simulink model "simulation_basic"  (R2022b)
settings: Solver=ode4  StartTime=0.0  StopTime=10  FixedStep=5e-7  MaxStep=1e-6  RelTol=1e-3
undefined symbols (not defined in the file or in its folder): current, Down, inverter, motor, speed, Up
libraries: simulink x11, eeGeneralControl x7, mcbcontrolslib x5, slpidlib x3, SignalEditorBlockLib x2, spsTriangleGeneratorLib x2, spsSampleandHoldLib x1
(part 1 of 2)
settings Model: Creator=Rizwan Sadik  LastModifiedBy=Rizwan Sadik
settings DataIOCC: SaveOutput=off  SaveTime=off

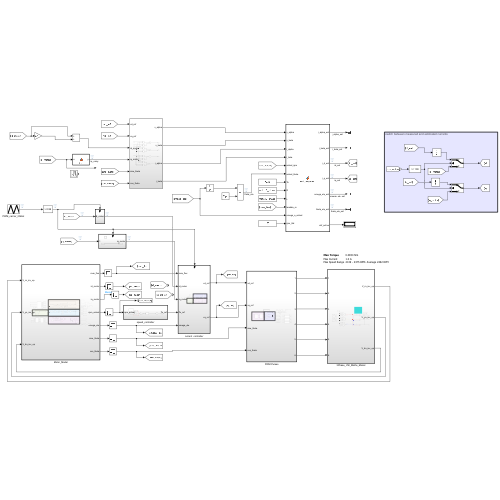
[thumbnail: Simulink's stored preview of the top-level diagram]
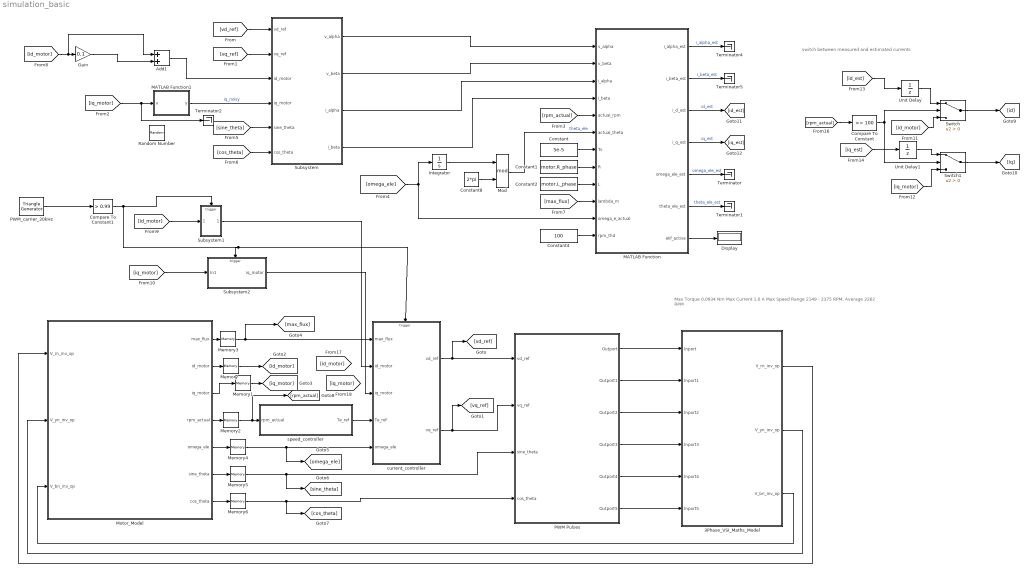
== system simulation_basic ==
  note: switch between measured and estimated currents
  note: Max Torque
      | 0.0934 Nm
      |
      | Max Current
      | 1.0 A
      |
      | Max Speed Range
      | 2149 - 2375 RPM. Average 2262 RPM
  3Phase_VSI_Maths_Model : Subsystem  Description=|  TreatAsAtomicUnit=on
      | Input DC Voltage = Vdc
      | Ouput Phase Voltages = Vrn, Vyn, Vbn
      | 
      | Pole Voltage = Vdc/2
      | Pole Voltages - instantaneous values:
      | Vro = +- Vdc/2
      | Vyo = +- Vdc/2
      | Vbo = +- Vdc/2
      | 
      | Leg 1 o/p is Vr. Switches 1 & 4
      | sw 1 ON (sw 4 OFF) -> Vro = +Vdc/2
      | sw 4 ON (sw 1 OFF) -> Vro = -Vdc/2
      | 
      | Leg 2 o/p is Vy. Switches 3 & 6
      | sw 3 ON (sw 6 OFF) -> Vyo = +Vdc/2
      | sw 6 ON (sw 3 OFF) -> Vyo = -Vdc/2
      | 
      | Leg 3 o/p is Vb. Switches 5 & 2
      | sw 5 ON (sw 2 OFF) -> Vbo = +Vdc/2
      | sw 2 ON (sw 5 OFF) -> Vbo = -Vdc/2
      | 
      | Vrn = (2Vro-Vyo-Vbo)/3
      | Vyn = (2Vyo-Vro-Vbo)/3
      | Vbn =(2Vbo-Vyo-Vro)/3
  Add1 : Sum
  Compare To Constant : simulink/Logic and Bit Operations/Compare To Constant  relop=>=  const=100  OutDataTypeStr=boolean
  Compare To Constant1 : simulink/Logic and Bit Operations/Compare To Constant  relop=>  const=0.99  OutDataTypeStr=boolean
  Constant : Constant  Value=5e-5
  Constant1 : Constant  Value=motor.R_phase
  Constant2 : Constant  Value=motor.L_phase
  Constant4 : Constant  Value=100
  Constant8 : Constant  Value=2*pi
  Display : Display
  Gain : Gain  Gain=0.1
  Integrator : Integrator  WrappedStateUpperValue=2*pi  WrappedStateLowerValue=0
  MATLAB Function : MATLAB Function  TreatAsAtomicUnit=on
  MATLAB Function1 : MATLAB Function  TreatAsAtomicUnit=on
  Memory{,1..6} (7 alike) : Memory
  Mod : Math  Operator=mod
  Motor_Model : Subsystem  TreatAsAtomicUnit=on
  PWM Pulses : Subsystem  TreatAsAtomicUnit=on
  PWM_carrier_20kHz : spsTriangleGeneratorLib/Triangle Generator  Freq=20000  Phase=0  Ts=0
  Random Number : RandomNumber  SampleTime=0.1
  Subsystem : Subsystem
  Subsystem1 : Subsystem
  Subsystem2 : Subsystem
  Switch : Switch  Criteria=u2 > Threshold  SaturateOnIntegerOverflow=off  InputSameDT=off
  Switch1 : Switch  Criteria=u2 > Threshold  SaturateOnIntegerOverflow=off  InputSameDT=off
  Terminator{,1..2,4..5} (5 alike) : Terminator
  Unit Delay : UnitDelay  SampleTime=-1  HasFrameUpgradeWarning=on
  Unit Delay1 : UnitDelay  SampleTime=-1  HasFrameUpgradeWarning=on
  current_controller : Subsystem  TreatAsAtomicUnit=on
  speed_controller : Subsystem  TreatAsAtomicUnit=on
  wires:
  speed_controller/1(Te_ref) -> current_controller/4(Te_ref)
  PWM Pulses/1(Outport) -> 3Phase_VSI_Maths_Model/1(Inport)
  Motor_Model/1(max_flux) -> Memory3/1
  PWM Pulses/4(Outport3) -> 3Phase_VSI_Maths_Model/4(Inport3)
  PWM Pulses/5(Outport4) -> 3Phase_VSI_Maths_Model/5(Inport4)
  Motor_Model/6(sine_theta) -> Memory5/1
  PWM Pulses/3(Outport2) -> 3Phase_VSI_Maths_Model/3(Inport2)
  Motor_Model/3(iq_motor) -> Memory1/1
  PWM Pulses/2(Outport1) -> 3Phase_VSI_Maths_Model/2(Inport1)
  PWM Pulses/6(Outport5) -> 3Phase_VSI_Maths_Model/6(Inport5)
  Motor_Model/2(id_motor) -> Memory/1
  Motor_Model/7(cos_theta) -> Memory6/1
  current_controller/2(vq_ref) -> [vq_ref], PWM Pulses/2(vq_ref)
  current_controller/1(vd_ref) -> [vd_ref], PWM Pulses/1(vd_ref)
  3Phase_VSI_Maths_Model/3(V_bn_inv_op) -> Motor_Model/3(V_bn_inv_op)
  3Phase_VSI_Maths_Model/2(V_yn_inv_op) -> Motor_Model/2(V_yn_inv_op)
  3Phase_VSI_Maths_Model/1(V_rn_inv_op) -> Motor_Model/1(V_rn_inv_op)
  Motor_Model/4(rpm_actual) -> Memory2/1
  Subsystem/3(i_alpha) -> MATLAB Function/3(i_alpha)
  Subsystem/4(i_beta) -> MATLAB Function/4(i_beta)
  Constant/1 -> MATLAB Function/7(Ts)
  Constant1/1 -> MATLAB Function/8(R)
  Constant2/1 -> MATLAB Function/9(L)
  MATLAB Function/5(omega_ele_est) -> Terminator/1  "omega_ele_est"
  MATLAB Function/6(theta_ele_est) -> Terminator1/1  "theta_ele_est"
  Motor_Model/5(omega_ele) -> Memory4/1
  Constant4/1 -> MATLAB Function/12(rpm_thd)
  MATLAB Function/7(ekf_active) -> Display/1
  Mod/1 -> MATLAB Function/6(actual_theta)  "theta_ele"
  Constant8/1 -> Mod/2
  Integrator/1 -> Mod/1
  Subsystem/1(v_alpha) -> MATLAB Function/1(v_alpha)
  Subsystem/2(v_beta) -> MATLAB Function/2(v_beta)
  [omega_ele] -> MATLAB Function/11(omega_e_actual), Integrator/1
  MATLAB Function/3(i_d_est) -> [id_est]  "id_est"
  MATLAB Function/4(i_q_est) -> [iq_est]  "iq_est"
  [vd_ref] -> Subsystem/1(vd_ref)
  [vq_ref] -> Subsystem/2(vq_ref)
  [id_motor] -> Add1/1, Gain/1
  [iq_motor] -> Terminator2/1, MATLAB Function1/1(u)
  [sine_theta] -> Subsystem/5(sine_theta)
  [cos_theta] -> Subsystem/6(cos_theta)
  [max_flux] -> MATLAB Function/10(lambda_m)
  [rpm_actual] -> MATLAB Function/5(actual_rpm)
  MATLAB Function/2(i_beta_est) -> Terminator5/1  "i_beta_est"
  MATLAB Function/1(i_alpha_est) -> Terminator4/1  "i_alpha_est"
  Subsystem1/1(id_motor) -> current_controller/2(id_motor)
  Subsystem2/1(iq_motor) -> current_controller/3(iq_motor)
  Switch/1 -> [id]
  Switch1/1 -> [iq]
  [id_motor] -> Switch/3
  [iq_motor] -> Switch1/3
  [id_est] -> Unit Delay/1
  [iq_est] -> Unit Delay1/1
  [rpm_actual] -> Compare To Constant/1
  Compare To Constant/1 -> Switch1/2, Switch/2
  Unit Delay/1 -> Switch/1
  Unit Delay1/1 -> Switch1/1
  Memory/1 -> [id_motor]
  Memory1/1 -> [iq_motor]
  Memory2/1 -> [rpm_actual], speed_controller/1(rpm_actual)
  Memory3/1 -> [max_flux], current_controller/1(max_flux)
  Memory4/1 -> [omega_ele], current_controller/5(omega_ele)
  Memory5/1 -> [sine_theta], PWM Pulses/3(sine_theta)
  Memory6/1 -> [cos_theta], PWM Pulses/4(cos_theta)
  Gain/1 -> Add1/2
  Add1/1 -> Subsystem/3(id_motor)
  MATLAB Function1/1(y) -> Subsystem/4(iq_motor)  "iq_noisy"
  PWM_carrier_20kHz/1 -> Compare To Constant1/1
  Compare To Constant1/1 -> current_controller/Trigger, Subsystem2/Trigger, Subsystem1/Trigger
  [id_motor] -> Subsystem1/1(In1)
  [iq_motor] -> Subsystem2/1(In1)

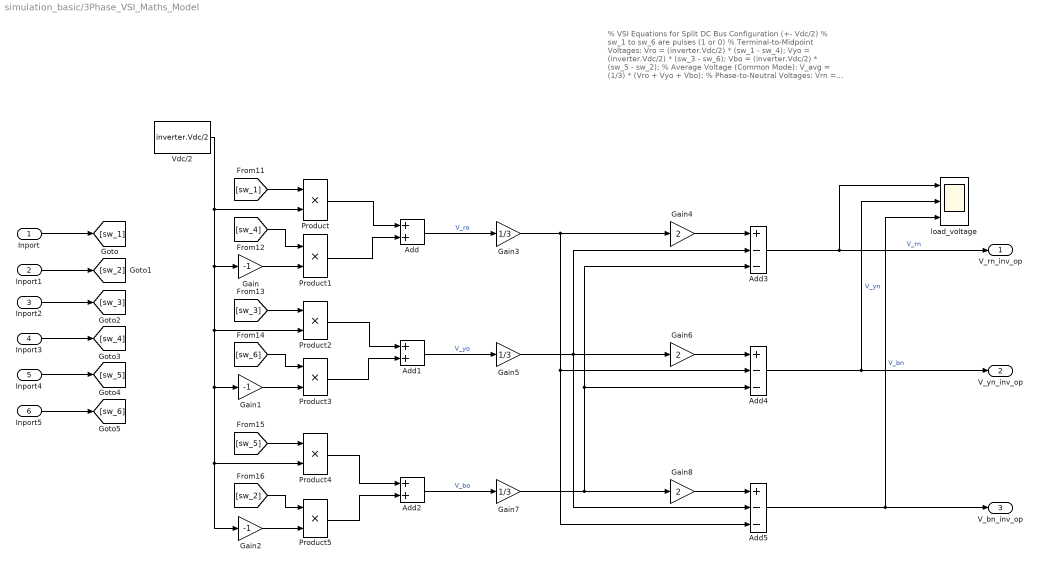
== system simulation_basic/3Phase_VSI_Maths_Model ==
  note: % VSI Equations for Split DC Bus Configuration (+- Vdc/2)
      | % sw_1 to sw_6 are pulses (1 or 0)
      |
      | % Terminal-to-Midpoint Voltages:
      | Vro = (inverter.Vdc/2) * (sw_1 - sw_4);
      | Vyo = (inverter.Vdc/2) * (sw_3 - sw_6);
      | Vbo = (inverter.Vdc/2) * (sw_5 - sw_2);
      |
      | % Average Voltage (Common Mode):
      | V_avg = (1/3) * (Vro + Vyo + Vbo);
      |
      | % Phase-to-Neutral Voltages:
      | Vrn = Vro - V_avg;
      | Vyn = Vyo - V_avg;
      | Vbn = Vbo - V_avg;
  Inport : Inport
  Inport1 : Inport  Port=2
  Inport2 : Inport  Port=3
  Inport3 : Inport  Port=4
  Inport4 : Inport  Port=5
  Inport5 : Inport  Port=6
  Add : Sum
  Add1 : Sum
  Add2 : Sum
  Add3 : Sum  Inputs=+--
  Add4 : Sum  Inputs=+--
  Add5 : Sum  Inputs=+--
  Gain : Gain  Gain=-1
  Gain1 : Gain  Gain=-1
  Gain2 : Gain  Gain=-1
  Gain3 : Gain  Gain=1/3
  Gain4 : Gain  Gain=2
  Gain5 : Gain  Gain=1/3
  Gain6 : Gain  Gain=2
  Gain7 : Gain  Gain=1/3
  Gain8 : Gain  Gain=2
  Product{,1..5} (6 alike) : Product
  Vdc/2 : Constant  Value=inverter.Vdc/2
  load_voltage : Scope  NumInputPorts=3
  V_rn_inv_op : Outport
  V_yn_inv_op : Outport  Port=2
  V_bn_inv_op : Outport  Port=3
  wires:
  Product2/1 -> Add1/1
  Add3/1 -> load_voltage/1, V_rn_inv_op/1  "V_rn"
  Product/1 -> Add/1
  Product4/1 -> Add2/1
  Vdc/2/1 -> Gain2/1, Product4/2, Gain1/1, Product2/2, Gain/1, Product/2
  Gain3/1 -> Add5/3, Add4/2, Gain4/1
  Add4/1 -> load_voltage/2, V_yn_inv_op/1  "V_yn"
  [sw_5] -> Product4/1
  Add/1 -> Gain3/1  "V_ro"
  Gain8/1 -> Add5/1
  Add2/1 -> Gain7/1  "V_bo"
  Gain7/1 -> Gain8/1, Add3/3, Add4/3
  Product5/1 -> Add2/2
  Gain5/1 -> Add5/2, Gain6/1, Add3/2
  [sw_3] -> Product2/1
  Gain4/1 -> Add3/1
  [sw_6] -> Product3/1
  Product3/1 -> Add1/2
  [sw_2] -> Product5/1
  Gain1/1 -> Product3/2
  Gain/1 -> Product1/2
  Product1/1 -> Add/2
  [sw_4] -> Product1/1
  [sw_1] -> Product/1
  Gain2/1 -> Product5/2
  Gain6/1 -> Add4/1
  Add5/1 -> V_bn_inv_op/1, load_voltage/3  "V_bn"
  Inport/1 -> [sw_1]
  Inport1/1 -> [sw_2]
  Inport3/1 -> [sw_4]
  Inport2/1 -> [sw_3]
  Inport5/1 -> [sw_6]
  Inport4/1 -> [sw_5]
  Add1/1 -> Gain5/1  "V_yo"

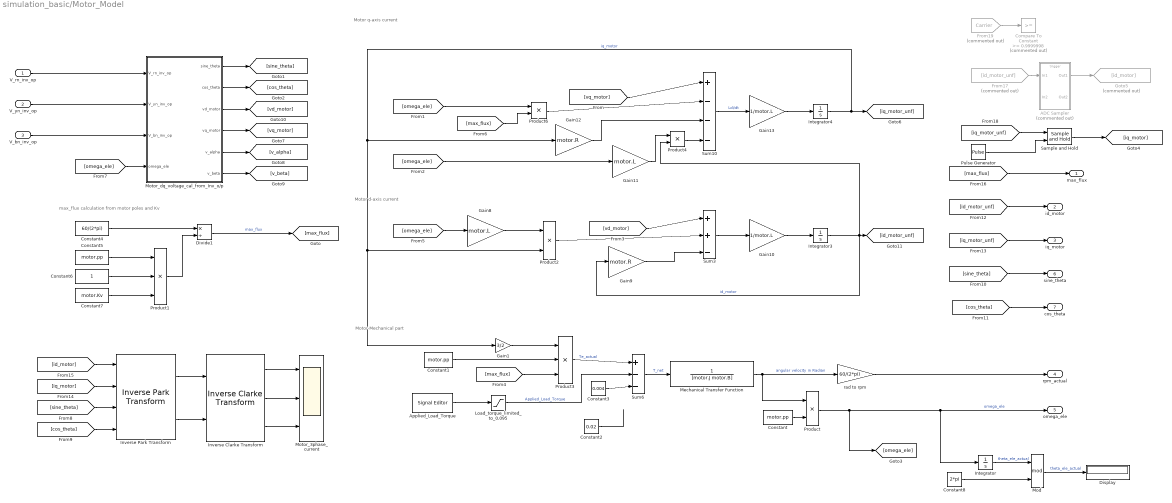
== system simulation_basic/Motor_Model ==
  note: max_flux calculation from motor poles and Kv
  note: Motor-Mechanical part
  note: Motor d-axis current
  note: Motor q-axis current
  V_rn_inv_op : Inport
  V_yn_inv_op : Inport  Port=2
  V_bn_inv_op : Inport  Port=3
  ADC Sampler : Subsystem  Commented=on
  Applied_Load_Torque : SignalEditorBlockLib/Signal Editor  FileName=signal_editor.mat  ActiveScenario=Scenario  ActiveSignal=1  IsBus=off  OutputBusObjectStr=Bus: BusObject  SampleTime=0  ZeroCross=off  OutputAfterFinalValue=Setting to zero  Unit=inherit  PreserveSignalName=on
  Compare To Constant : simulink/Logic and Bit Operations/Compare To Constant  Commented=on  relop=>=  const=0.9999998  OutDataTypeStr=boolean
  Constant : Constant  Value=motor.pp
  Constant1 : Constant  Value=motor.pp
  Constant2 : Constant  Value=0.02
  Constant3 : Constant  Value=0.004
  Constant4 : Constant  Value=60/(2*pi)
  Constant5 : Constant  Value=motor.pp
  Constant6 : Constant
  Constant7 : Constant  Value=motor.Kv
  Constant8 : Constant  Value=2*pi
  Display : Display
  Divide1 : Product  Inputs=*/
  From17 : From  Commented=on  GotoTag=id_motor_unf
  From19 : From  Commented=on  GotoTag=Carrier  TagVisibility=global
  Gain1 : Gain  Gain=3/2
  Gain10 : Gain  Gain=1/motor.L
  Gain11 : Gain  Gain=motor.L
  Gain12 : Gain  Gain=motor.R
  Gain13 : Gain  Gain=1/motor.L
  Gain8 : Gain  Gain=motor.L
  Gain9 : Gain  Gain=motor.R
  Goto5 : Goto  Commented=on  GotoTag=id_motor
  Integrator : Integrator  WrappedStateUpperValue=2*pi  WrappedStateLowerValue=0
  Integrator3 : Integrator
  Integrator4 : Integrator
  Inverse Clarke Transform : mcbcontrolslib/Inverse Clarke Transform
      settings: LibrarySourceBlock=mcbhdllib/Controls/Math Transforms/Inverse Clarke Transform
  Inverse Park Transform : mcbcontrolslib/Inverse Park Transform  AxisAlignment=D-axis
      settings: LibrarySourceBlock=mcblib/Controls/Math Transforms/Inverse Park Transform
  Load_torque_limited_to_0.095 : Saturate  UpperLimit=0.095  LowerLimit=0
  Mechanical Transfer Function : TransferFcn  Denominator=[motor.J motor.B]
  Mod : Math  Operator=mod
  Motor_3phase_current : Scope  NumInputPorts=3
  Motor_dq_voltage_cal_from_Inv_o/p : Subsystem
  Product{,2,4,6} (4 alike) : Product
  Product1 : Product  Inputs=3
  Product3 : Product  Inputs=3
  Pulse Generator : DiscretePulseGenerator  Period=100  SampleTime=5e-7
  Sample and Hold : spsSampleandHoldLib/Sample and Hold  ic=0  Ts=0
      settings: LibrarySourceBlock=|
      | sps_lib/Control/Sample and
      | Hold
  Sum10 : Sum  Inputs=|+---
  Sum3 : Sum  Inputs=|++-
  Sum6 : Sum  Inputs=+|--
  rad to rpm : Gain  Gain=60/(2*pi)
  max_flux : Outport
  id_motor : Outport  Port=2
  iq_motor : Outport  Port=3
  rpm_actual : Outport  Port=4
  omega_ele : Outport  Port=5
  sine_theta : Outport  Port=6
  cos_theta : Outport  Port=7
  wires:
  Product6/1 -> Sum10/2
  Gain12/1 -> Sum10/3
  [max_flux] -> Product6/2
  Gain13/1 -> Integrator4/1
  Gain11/1 -> Product4/1
  Integrator4/1 -> [iq_motor_unf], Gain1/1, Product2/2, Gain12/1  "iq_motor"
  Product4/1 -> Sum10/4
  [omega_ele] -> Gain11/1
  Sum10/1 -> Gain13/1  "Ldi/dt​​"
  [vq_motor] -> Sum10/1
  [omega_ele] -> Product6/1
  Product2/1 -> Sum3/2
  Integrator3/1 -> [id_motor_unf], Gain9/1, Product4/2  "id_motor"
  Gain9/1 -> Sum3/3
  Gain8/1 -> Product2/1
  Sum3/1 -> Gain10/1
  Gain10/1 -> Integrator3/1
  [omega_ele] -> Gain8/1
  [vd_motor] -> Sum3/1
  [max_flux] -> Product3/3
  Constant/1 -> Product/2
  Mechanical Transfer Function/1 -> rad to rpm/1, Product/1  "angular velocity in Radian"
  Sum6/1 -> Mechanical Transfer Function/1  "T_net"
  Constant3/1 -> Sum6/3
  Gain1/1 -> Product3/1
  Product3/1 -> Sum6/1  "Te_actual"
  Load_torque_limited_to_0.095/1 -> Sum6/2  "Applied_Load_Torque"
  Constant1/1 -> Product3/2
  rad to rpm/1 -> rpm_actual/1
  Constant6/1 -> Product1/2
  Product1/1 -> Divide1/2
  Constant5/1 -> Product1/1
  Constant7/1 -> Product1/3
  Constant4/1 -> Divide1/1
  Divide1/1 -> [max_flux]  "max_flux"
  Applied_Load_Torque/1 -> Load_torque_limited_to_0.095/1
  V_rn_inv_op/1 -> Motor_dq_voltage_cal_from_Inv_o/p/1(V_rn_inv_op)
  V_yn_inv_op/1 -> Motor_dq_voltage_cal_from_Inv_o/p/2(V_yn_inv_op)
  V_bn_inv_op/1 -> Motor_dq_voltage_cal_from_Inv_o/p/3(V_bn_inv_op)
  [omega_ele] -> Motor_dq_voltage_cal_from_Inv_o/p/4(omega_ele)
  Motor_dq_voltage_cal_from_Inv_o/p/2(cos_theta) -> [cos_theta]
  Motor_dq_voltage_cal_from_Inv_o/p/3(vd_motor) -> [vd_motor]
  Motor_dq_voltage_cal_from_Inv_o/p/4(vq_motor) -> [vq_motor]
  Inverse Clarke Transform/2 -> Motor_3phase_current/2
  Inverse Clarke Transform/1 -> Motor_3phase_current/1
  Inverse Park Transform/1 -> Inverse Clarke Transform/1
  Inverse Clarke Transform/3 -> Motor_3phase_current/3
  Inverse Park Transform/2 -> Inverse Clarke Transform/2
  Motor_dq_voltage_cal_from_Inv_o/p/1(sine_theta) -> [sine_theta]
  [sine_theta] -> Inverse Park Transform/3
  [cos_theta] -> Inverse Park Transform/4
  [sine_theta] -> sine_theta/1
  [cos_theta] -> cos_theta/1
  [id_motor_unf] -> id_motor/1
  [iq_motor_unf] -> iq_motor/1
  [iq_motor] -> Inverse Park Transform/2
  [id_motor] -> Inverse Park Transform/1
  [max_flux] -> max_flux/1
  Constant2/1 -> ?
  Product/1 -> [omega_ele], omega_ele/1, Integrator/1  "omega_ele"
  Mod/1 -> Display/1  "theta_ele_actual"
  Constant8/1 -> Mod/2
  Integrator/1 -> Mod/1  "theta_ele_actual"
  Motor_dq_voltage_cal_from_Inv_o/p/5(v_alpha) -> [v_alpha]
  Motor_dq_voltage_cal_from_Inv_o/p/6(v_beta) -> [v_beta]
  From17/1 -> ADC Sampler/1(In1)
  [iq_motor_unf] -> Sample and Hold/1
  ADC Sampler/1(Out1) -> Goto5/1
  From19/1 -> Compare To Constant/1
  Sample and Hold/1 -> [iq_motor]
  Pulse Generator/1 -> Sample and Hold/2

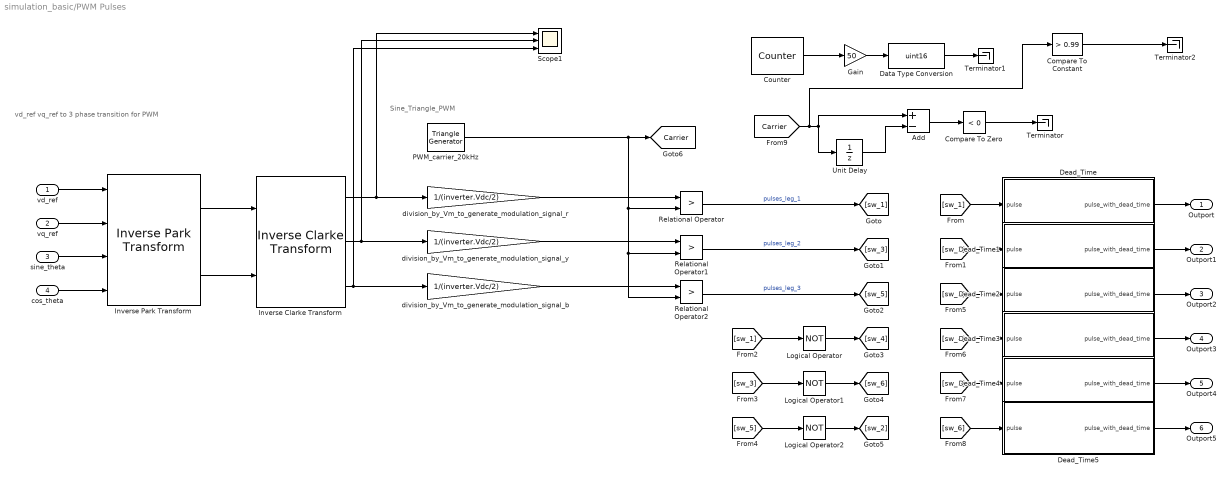
== system simulation_basic/PWM Pulses ==
  note: vd_ref vq_ref to 3 phase transition for PWM
  note: Sine_Triangle_PWM
  vd_ref : Inport
  vq_ref : Inport  Port=2
  sine_theta : Inport  Port=3
  cos_theta : Inport  Port=4
  Add : Sum  Inputs=+-
  Compare To Constant : simulink/Logic and Bit Operations/Compare To Constant  relop=>  const=0.99  OutDataTypeStr=boolean
  Compare To Zero : simulink/Logic and Bit Operations/Compare To Zero  relop=<  OutDataTypeStr=boolean
  Counter : eeGeneralControl/Counter  CarrCount=Up-Down  Range=[0 1]  Tper=2.5e-5  Tdelay=0  Ts=5e-7
      settings: LibrarySourceBlock=ee_sl_lib/General Control/Counter
  Data Type Conversion : DataTypeConversion  OutDataTypeStr=uint16  SaturateOnIntegerOverflow=off  RndMeth=Floor
  Dead_Time : Subsystem
  Dead_Time1 : Subsystem
  Dead_Time2 : Subsystem
  Dead_Time3 : Subsystem
  Dead_Time4 : Subsystem
  Dead_Time5 : Subsystem
  Gain : Gain  Gain=50
  Inverse Clarke Transform : mcbcontrolslib/Inverse Clarke Transform
      settings: LibrarySourceBlock=mcbhdllib/Controls/Math Transforms/Inverse Clarke Transform
  Inverse Park Transform : mcbcontrolslib/Inverse Park Transform  AxisAlignment=D-axis
      settings: LibrarySourceBlock=mcblib/Controls/Math Transforms/Inverse Park Transform
  Logical Operator : Logic  Operator=NOT  AllPortsSameDT=off  OutDataTypeStr=boolean
  Logical Operator1 : Logic  Operator=NOT  AllPortsSameDT=off  OutDataTypeStr=boolean
  Logical Operator2 : Logic  Operator=NOT  AllPortsSameDT=off  OutDataTypeStr=boolean
  PWM_carrier_20kHz : spsTriangleGeneratorLib/Triangle Generator  Freq=20000  Phase=0  Ts=0
  Relational Operator : RelationalOperator  Operator=>  OutDataTypeStr=boolean  RndMeth=Simplest  InputSameDT=off
  Relational Operator1 : RelationalOperator  Operator=>  OutDataTypeStr=boolean  RndMeth=Simplest  InputSameDT=off
  Relational Operator2 : RelationalOperator  Operator=>  OutDataTypeStr=boolean  RndMeth=Simplest  InputSameDT=off
  Scope1 : Scope  NumInputPorts=3
  Terminator : Terminator
  Terminator1 : Terminator
  Terminator2 : Terminator
  Unit Delay : UnitDelay  SampleTime=-1  HasFrameUpgradeWarning=on
  division_by_Vm_to_generate_modulation_signal_b : Gain  Gain=1/(inverter.Vdc/2)
  division_by_Vm_to_generate_modulation_signal_r : Gain  Gain=1/(inverter.Vdc/2)
  division_by_Vm_to_generate_modulation_signal_y : Gain  Gain=1/(inverter.Vdc/2)
  Outport : Outport
  Outport1 : Outport  Port=2
  Outport2 : Outport  Port=3
  Outport3 : Outport  Port=4
  Outport4 : Outport  Port=5
  Outport5 : Outport  Port=6
  tag scope: Carrier=global
  wires:
  [sw_3] -> Logical Operator1/1
  Logical Operator2/1 -> [sw_2]
  cos_theta/1 -> Inverse Park Transform/4
  sine_theta/1 -> Inverse Park Transform/3
  [sw_5] -> Logical Operator2/1
  Inverse Park Transform/2 -> Inverse Clarke Transform/2
  Inverse Park Transform/1 -> Inverse Clarke Transform/1
  Logical Operator/1 -> [sw_4]
  Logical Operator1/1 -> [sw_6]
  [sw_1] -> Logical Operator/1
  vd_ref/1 -> Inverse Park Transform/1
  vq_ref/1 -> Inverse Park Transform/2
  [sw_1] -> Dead_Time/1(pulse)
  [sw_6] -> Dead_Time5/1(pulse)
  [sw_2] -> Dead_Time1/1(pulse)
  [sw_3] -> Dead_Time2/1(pulse)
  [sw_4] -> Dead_Time3/1(pulse)
  [sw_5] -> Dead_Time4/1(pulse)
  Relational Operator2/1 -> [sw_5]  "pulses_leg_3"
  Relational Operator1/1 -> [sw_3]  "pulses_leg_2"
  Relational Operator/1 -> [sw_1]  "pulses_leg_1"
  PWM_carrier_20kHz/1 -> [Carrier], Relational Operator2/2, Relational Operator1/2, Relational Operator/2
  division_by_Vm_to_generate_modulation_signal_y/1 -> Relational Operator1/1
  division_by_Vm_to_generate_modulation_signal_b/1 -> Relational Operator2/1
  Inverse Clarke Transform/3 -> Scope1/3, division_by_Vm_to_generate_modulation_signal_b/1
  Inverse Clarke Transform/2 -> Scope1/2, division_by_Vm_to_generate_modulation_signal_y/1
  division_by_Vm_to_generate_modulation_signal_r/1 -> Relational Operator/1
  Inverse Clarke Transform/1 -> Scope1/1, division_by_Vm_to_generate_modulation_signal_r/1
  Dead_Time/1(pulse_with_dead_time) -> Outport/1
  Dead_Time1/1(pulse_with_dead_time) -> Outport1/1
  Dead_Time2/1(pulse_with_dead_time) -> Outport2/1
  Dead_Time3/1(pulse_with_dead_time) -> Outport3/1
  Dead_Time4/1(pulse_with_dead_time) -> Outport4/1
  Dead_Time5/1(pulse_with_dead_time) -> Outport5/1
  [Carrier] -> Compare To Constant/1, Unit Delay/1, Add/1
  Unit Delay/1 -> Add/2
  Add/1 -> Compare To Zero/1
  Counter/1 -> Gain/1
  Compare To Zero/1 -> Terminator/1
  Gain/1 -> Data Type Conversion/1
  Data Type Conversion/1 -> Terminator1/1
  Compare To Constant/1 -> Terminator2/1

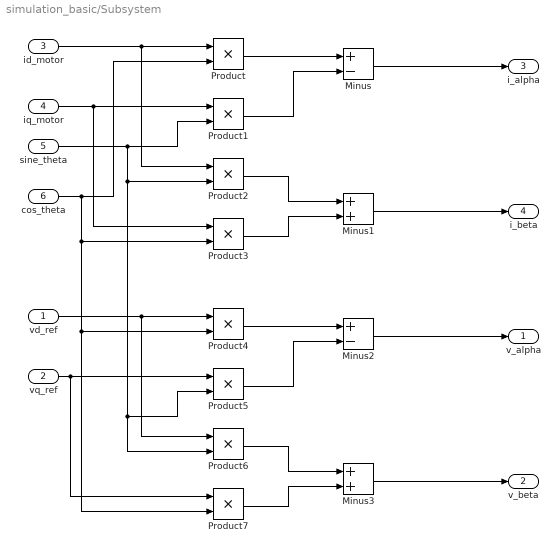
== system simulation_basic/Subsystem ==
  vd_ref : Inport
  vq_ref : Inport  Port=2
  id_motor : Inport  Port=3
  iq_motor : Inport  Port=4
  sine_theta : Inport  Port=5
  cos_theta : Inport  Port=6
  Minus : Sum  Inputs=+-
  Minus1 : Sum
  Minus2 : Sum  Inputs=+-
  Minus3 : Sum
  Product{,1..7} (8 alike) : Product
  v_alpha : Outport
  v_beta : Outport  Port=2
  i_alpha : Outport  Port=3
  i_beta : Outport  Port=4
  wires:
  id_motor/1 -> Product2/1, Product/1
  iq_motor/1 -> Product3/1, Product1/1
  Product/1 -> Minus/1
  Product1/1 -> Minus/2
  Minus/1 -> i_alpha/1
  Product2/1 -> Minus1/1
  Product3/1 -> Minus1/2
  Minus1/1 -> i_beta/1
  Minus3/1 -> v_beta/1
  Product7/1 -> Minus3/2
  Product6/1 -> Minus3/1
  Minus2/1 -> v_alpha/1
  Product5/1 -> Minus2/2
  sine_theta/1 -> Product5/2, Product6/2, Product2/2, Product1/2
  Product4/1 -> Minus2/1
  cos_theta/1 -> Product7/2, Product4/2, Product3/2, Product/2
  vq_ref/1 -> Product5/1, Product7/1
  vd_ref/1 -> Product4/1, Product6/1

== system simulation_basic/Subsystem1 ==
  In1 : Inport
  Trigger : TriggerPort  VariantControl=(inherit)  PortDimensions=1
  id_motor : Outport
  wires:
  In1/1 -> id_motor/1

== system simulation_basic/Subsystem2 ==
  In1 : Inport
  Trigger : TriggerPort  VariantControl=(inherit)  PortDimensions=1
  iq_motor : Outport
  wires:
  In1/1 -> iq_motor/1

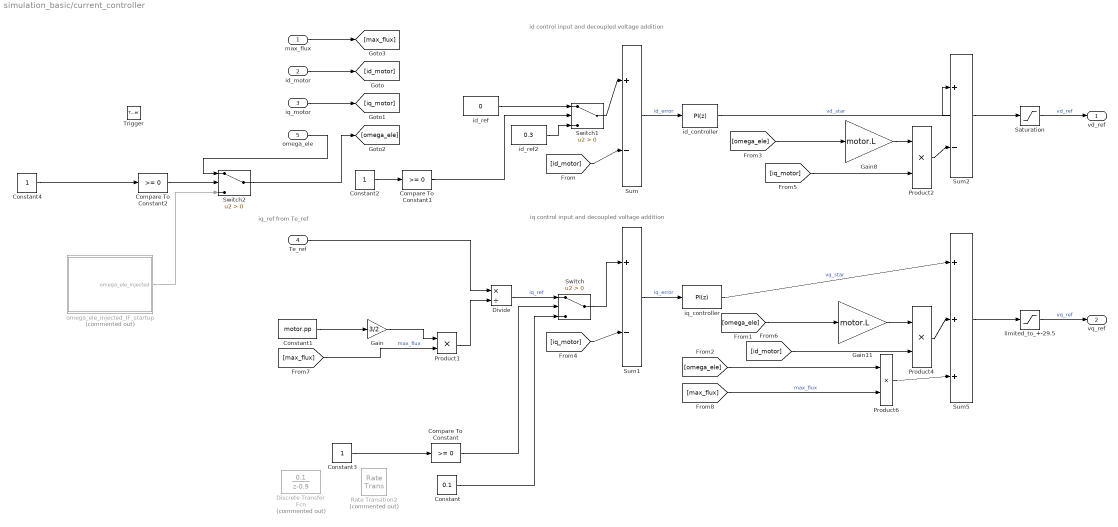
== system simulation_basic/current_controller ==
  note: iq_ref from Te_ref
  note: iq control input and decoupled voltage addition
  note: id control input and decoupled voltage addition
  max_flux : Inport
  id_motor : Inport  Port=2
  iq_motor : Inport  Port=3
  Te_ref : Inport  Port=4
  omega_ele : Inport  Port=5
  Trigger : TriggerPort  VariantControl=(inherit)  PortDimensions=1
  Compare To Constant : simulink/Logic and Bit Operations/Compare To Constant  relop=>=  const=0  OutDataTypeStr=boolean
  Compare To Constant1 : simulink/Logic and Bit Operations/Compare To Constant  relop=>=  const=0  OutDataTypeStr=boolean
  Compare To Constant2 : simulink/Logic and Bit Operations/Compare To Constant  relop=>=  const=0  OutDataTypeStr=boolean
  Constant : Constant  Value=0.1
  Constant1 : Constant  Value=motor.pp
  Constant2 : Constant
  Constant3 : Constant
  Constant4 : Constant
  Discrete Transfer Fcn : DiscreteTransferFcn  Commented=on  Numerator=[0.1]  Denominator=[1 -0.9]  SampleTime=5e-5
  Divide : Product  Inputs=*/
  Gain : Gain  Gain=3/2
  Gain11 : Gain  Gain=motor.L
  Gain8 : Gain  Gain=motor.L
  Product{1..2,4,6} (4 alike) : Product
  Rate Transition2 : RateTransition  Commented=on  Integrity=off  OutPortSampleTime=5e-5
  Saturation : Saturate  UpperLimit=29.5  LowerLimit=-29.5
  Sum : Sum  Inputs=|+-
  Sum1 : Sum  Inputs=|+-
  Sum2 : Sum  Inputs=|+-
  Sum5 : Sum  Inputs=|+++
  Switch : Switch  Criteria=u2 > Threshold  SaturateOnIntegerOverflow=off  InputSameDT=off
  Switch1 : Switch  Criteria=u2 > Threshold  SaturateOnIntegerOverflow=off  InputSameDT=off
  Switch2 : Switch  Criteria=u2 > Threshold  SaturateOnIntegerOverflow=off  InputSameDT=off
  id_controller : slpidlib/PID Controller  Controller=PI  Form=Parallel  TimeDomain=Discrete-time  UseExternalTs=off  SampleTime=-1  IntegratorMethod=Forward Euler  FilterMethod=Forward Euler  ControllerParametersSource=internal  P=current.Kp_id  I=current.Ki_id  UseKiTs=off  D=0  N=100  UseFilter=on  TunerSelectOption=Transfer Function Based (PID Tuner App)  InitialConditionSource=internal  InitialConditionForIntegrator=0  InitialConditionForFilter=0  DifferentiatorICPrevScaledInput=0  ExternalReset=none  TrackingMode=off  Kt=1  LimitOutput=on  SatLimitsSource=internal  UpperSaturationLimit=inf  LowerSaturationLimit=-inf  LinearizeAsGain=on  AntiWindupMode=clamping  Kb=1  LimitIntegrator=off  UpperIntegratorSaturationLimit=inf  LowerIntegratorSaturationLimit=-inf  POutMin=[]  POutMax=[]  IOutMin=[]  IOutMax=[]  DOutMin=[]  DOutMax=[]  NOutMin=[]  NOutMax=[]  SumOutMin=[]  SumOutMax=[]  SaturationOutMin=[]  SaturationOutMax=[]  PParamMin=[]  PParamMax=[]  IParamMin=[]  IParamMax=[]  DParamMin=[]  DParamMax=[]  NParamMin=[]  NParamMax=[]  KbParamMin=[]  KbParamMax=[]  KtParamMin=[]  KtParamMax=[]  KbOutMin=[]  KbOutMax=[]  KtOutMin=[]  KtOutMax=[]  IntegratorOutMin=[]  IntegratorOutMax=[]  FilterOutMin=[]  FilterOutMax=[]  SumI1OutMin=[]  SumI1OutMax=[]  SumI2OutMin=[]  SumI2OutMax=[]  SumI3OutMin=[]  SumI3OutMax=[]  SumI4OutMin=[]  SumI4OutMax=[]  SumDOutMin=[]  SumDOutMax=[]  DifferentiatorOutMin=[]  DifferentiatorOutMax=[]  FilterDiffOutCoefMin=[]  FilterDiffOutCoefMax=[]  ReciprocalOutMin=[]  ReciprocalOutMax=[]  SumDenOutMin=[]  SumDenOutMax=[]  SumNumOutMin=[]  SumNumOutMax=[]  DivideOutMin=[]  DivideOutMax=[]  UdiffTsProdOutMin=[]  UdiffTsProdOutMax=[]  NTsProdOutMin=[]  NTsProdOutMax=[]  UintegralTsProdOutMin=[]  UintegralTsProdOutMax=[]  UngainTsProdOutMin=[]  UngainTsProdOutMax=[]  ClampingZeroOutDataTypeStr=Inherit: Inherit via back propagation  ClampingZeroOutMin=[]  ClampingZeroOutMax=[]  FilterDenConstantOutDataTypeStr=Inherit: Inherit via back propagation  FilterDenConstantOutMin=[]  FilterDenConstantOutMax=[]  PCopyOutDataTypeStr=Inherit: Inherit via back propagation  PCopyOutMin=[]  PCopyOutMax=[]  NCopyOutDataTypeStr=Inherit: Inherit via back propagation  NCopyOutMin=[]  NCopyOutMax=[]  IntegratorContinuousStateAttributes=''  IntegratorStateMustResolveToSignalObject=off  IntegratorRTWStateStorageClass=Auto  FilterContinuousStateAttributes=''  FilterStateMustResolveToSignalObject=off  FilterRTWStateStorageClass=Auto  ParallelPVariant=InternalParameters  IdealPVariant=Disabled  IVariant=InternalParameters  DVariant=Disabled  IntegratorVariant=Discrete  SatVariant=Enabled  AWVariant=DiscClampingParallel  PCopyVariant=Disabled  TRVariant=Disabled  FdbkBlocksVariant=Forward  IdealPFdbkVariant=Disabled  SatFdbkVariant=Disabled  DerivativeFilterVariant=Disabled  NVariant=Disabled  NCopyVariant=Disabled_SignalSpec  FilterICVariant=Disabled  IntegratorICVariant=InternalICs  ExternalResetVariant=Disabled  TRSumVariant=Passthrough  SumFdbkVariant=Disabled  SumVariant=Sum_PI  TsampFilterVariant=InternalTs  TsampNgainVariant=Passthrough  TsampIntegralVariant=Passthrough  ExternalSaturationOutDataTypeStr=Inherit: Same as second input
  id_ref : Constant  Value=0
  id_ref2 : Constant  Value=0.3
  iq_controller : slpidlib/PID Controller  Controller=PI  Form=Parallel  TimeDomain=Discrete-time  UseExternalTs=off  SampleTime=-1  IntegratorMethod=Forward Euler  FilterMethod=Forward Euler  ControllerParametersSource=internal  P=current.Kp_iq  I=current.Ki_iq  UseKiTs=off  D=0  N=100  UseFilter=on  TunerSelectOption=Transfer Function Based (PID Tuner App)  InitialConditionSource=internal  InitialConditionForIntegrator=0  InitialConditionForFilter=0  DifferentiatorICPrevScaledInput=0  ExternalReset=none  TrackingMode=off  Kt=1  LimitOutput=on  SatLimitsSource=internal  UpperSaturationLimit=inf  LowerSaturationLimit=-inf  LinearizeAsGain=on  AntiWindupMode=clamping  Kb=1  LimitIntegrator=on  UpperIntegratorSaturationLimit=29.5  LowerIntegratorSaturationLimit=-29.5  POutMin=[]  POutMax=[]  IOutMin=[]  IOutMax=[]  DOutMin=[]  DOutMax=[]  NOutMin=[]  NOutMax=[]  SumOutMin=[]  SumOutMax=[]  SaturationOutMin=[]  SaturationOutMax=[]  PParamMin=[]  PParamMax=[]  IParamMin=[]  IParamMax=[]  DParamMin=[]  DParamMax=[]  NParamMin=[]  NParamMax=[]  KbParamMin=[]  KbParamMax=[]  KtParamMin=[]  KtParamMax=[]  KbOutMin=[]  KbOutMax=[]  KtOutMin=[]  KtOutMax=[]  IntegratorOutMin=[]  IntegratorOutMax=[]  FilterOutMin=[]  FilterOutMax=[]  SumI1OutMin=[]  SumI1OutMax=[]  SumI2OutMin=[]  SumI2OutMax=[]  SumI3OutMin=[]  SumI3OutMax=[]  SumI4OutMin=[]  SumI4OutMax=[]  SumDOutMin=[]  SumDOutMax=[]  DifferentiatorOutMin=[]  DifferentiatorOutMax=[]  FilterDiffOutCoefMin=[]  FilterDiffOutCoefMax=[]  ReciprocalOutMin=[]  ReciprocalOutMax=[]  SumDenOutMin=[]  SumDenOutMax=[]  SumNumOutMin=[]  SumNumOutMax=[]  DivideOutMin=[]  DivideOutMax=[]  UdiffTsProdOutMin=[]  UdiffTsProdOutMax=[]  NTsProdOutMin=[]  NTsProdOutMax=[]  UintegralTsProdOutMin=[]  UintegralTsProdOutMax=[]  UngainTsProdOutMin=[]  UngainTsProdOutMax=[]  ClampingZeroOutDataTypeStr=Inherit: Inherit via back propagation  ClampingZeroOutMin=[]  ClampingZeroOutMax=[]  FilterDenConstantOutDataTypeStr=Inherit: Inherit via back propagation  FilterDenConstantOutMin=[]  FilterDenConstantOutMax=[]  PCopyOutDataTypeStr=Inherit: Inherit via back propagation  PCopyOutMin=[]  PCopyOutMax=[]  NCopyOutDataTypeStr=Inherit: Inherit via back propagation  NCopyOutMin=[]  NCopyOutMax=[]  IntegratorContinuousStateAttributes=''  IntegratorStateMustResolveToSignalObject=off  IntegratorRTWStateStorageClass=Auto  FilterContinuousStateAttributes=''  FilterStateMustResolveToSignalObject=off  FilterRTWStateStorageClass=Auto  ParallelPVariant=InternalParameters  IdealPVariant=Disabled  IVariant=InternalParameters  DVariant=Disabled  IntegratorVariant=Discrete  SatVariant=Enabled  AWVariant=DiscClampingParallel  PCopyVariant=Disabled  TRVariant=Disabled  FdbkBlocksVariant=Forward  IdealPFdbkVariant=Disabled  SatFdbkVariant=Disabled  DerivativeFilterVariant=Disabled  NVariant=Disabled  NCopyVariant=Disabled_SignalSpec  FilterICVariant=Disabled  IntegratorICVariant=InternalICs  ExternalResetVariant=Disabled  TRSumVariant=Passthrough  SumFdbkVariant=Disabled  SumVariant=Sum_PI  TsampFilterVariant=InternalTs  TsampNgainVariant=Passthrough  TsampIntegralVariant=Passthrough  ExternalSaturationOutDataTypeStr=Inherit: Same as second input
  limited_to_+-29.5 : Saturate  UpperLimit=29.5  LowerLimit=-29.5
  omega_ele_injected_IF_startup : Subsystem  Commented=on
  vd_ref : Outport
  vq_ref : Outport  Port=2
  wires:
  Sum1/1 -> iq_controller/1  "iq_error"
  id_motor/1 -> [id_motor]
  Te_ref/1 -> Divide/1
  Sum5/1 -> limited_to_+-29.5/1
  Product4/1 -> Sum5/2
  Product6/1 -> Sum5/3
  iq_controller/1 -> Sum5/1  "vq_star"
  max_flux/1 -> [max_flux]
  Product2/1 -> Sum2/2
  Gain8/1 -> Product2/1
  Sum2/1 -> Saturation/1
  iq_motor/1 -> [iq_motor]
  id_controller/1 -> Sum2/1  "vd_star"
  Sum/1 -> id_controller/1  "id_error"
  Saturation/1 -> vd_ref/1  "vd_ref"
  [id_motor] -> Sum/2
  omega_ele/1 -> Switch2/1
  [omega_ele] -> Product6/1
  [iq_motor] -> Sum1/2
  Gain11/1 -> Product4/1
  Product1/1 -> Divide/2
  Gain/1 -> Product1/1
  Constant1/1 -> Gain/1
  [max_flux] -> Product1/2  "max_flux"
  [max_flux] -> Product6/2  "max_flux"
  [omega_ele] -> Gain8/1
  [iq_motor] -> Product2/2
  [id_motor] -> Product4/2
  [omega_ele] -> Gain11/1
  Constant3/1 -> Compare To Constant/1
  Compare To Constant/1 -> Switch/2
  Constant/1 -> Switch/3
  Switch/1 -> Sum1/1
  id_ref/1 -> Switch1/1
  id_ref2/1 -> Switch1/3
  Constant2/1 -> Compare To Constant1/1
  Compare To Constant1/1 -> Switch1/2
  Constant4/1 -> Compare To Constant2/1
  Compare To Constant2/1 -> Switch2/2
  omega_ele_injected_IF_startup/1(omega_ele_injected) -> Switch2/3
  Divide/1 -> Switch/1  "iq_ref"
  Switch1/1 -> Sum/1
  Switch2/1 -> [omega_ele]
  limited_to_+-29.5/1 -> vq_ref/1  "vq_ref"

== system simulation_basic/speed_controller ==
  rpm_actual : Inport
  Constant : Constant  Value=1000
  Sum2 : Sum  Inputs=|+-
  requested_torque_limited_to_0.1 : Saturate  UpperLimit=0.1  LowerLimit=-0.05
  rpm_ref : SignalEditorBlockLib/Signal Editor  FileName=signal_editor.mat  ActiveScenario=Scenario2  ActiveSignal=rpm_ramp  IsBus=off  OutputBusObjectStr=Bus: BusObject  SampleTime=0  ZeroCross=off  OutputAfterFinalValue=Setting to zero  Unit=inherit  PreserveSignalName=on
  rpm_to_rad/s : Gain  Gain=2*pi/60
  speed_controller : slpidlib/PID Controller  Controller=PI  Form=Parallel  TimeDomain=Discrete-time  UseExternalTs=off  SampleTime=1/2000  IntegratorMethod=Forward Euler  FilterMethod=Forward Euler  ControllerParametersSource=internal  P=speed.Kp_speed  I=speed.Ki_speed  UseKiTs=off  D=0  N=100  UseFilter=on  TunerSelectOption=Transfer Function Based (PID Tuner App)  InitialConditionSource=internal  InitialConditionForIntegrator=0  InitialConditionForFilter=0  DifferentiatorICPrevScaledInput=0  ExternalReset=none  TrackingMode=off  Kt=1  LimitOutput=on  SatLimitsSource=internal  UpperSaturationLimit=0.1  LowerSaturationLimit=-0.05  LinearizeAsGain=off  AntiWindupMode=clamping  Kb=1  LimitIntegrator=on  UpperIntegratorSaturationLimit=0.1  LowerIntegratorSaturationLimit=0  POutMin=[]  POutMax=[]  IOutMin=[]  IOutMax=[]  DOutMin=[]  DOutMax=[]  NOutMin=[]  NOutMax=[]  SumOutMin=[]  SumOutMax=[]  SaturationOutMin=[]  SaturationOutMax=[]  PParamMin=[]  PParamMax=[]  IParamMin=[]  IParamMax=[]  DParamMin=[]  DParamMax=[]  NParamMin=[]  NParamMax=[]  KbParamMin=[]  KbParamMax=[]  KtParamMin=[]  KtParamMax=[]  KbOutMin=[]  KbOutMax=[]  KtOutMin=[]  KtOutMax=[]  IntegratorOutMin=[]  IntegratorOutMax=[]  FilterOutMin=[]  FilterOutMax=[]  SumI1OutMin=[]  SumI1OutMax=[]  SumI2OutMin=[]  SumI2OutMax=[]  SumI3OutMin=[]  SumI3OutMax=[]  SumI4OutMin=[]  SumI4OutMax=[]  SumDOutMin=[]  SumDOutMax=[]  DifferentiatorOutMin=[]  DifferentiatorOutMax=[]  FilterDiffOutCoefMin=[]  FilterDiffOutCoefMax=[]  ReciprocalOutMin=[]  ReciprocalOutMax=[]  SumDenOutMin=[]  SumDenOutMax=[]  SumNumOutMin=[]  SumNumOutMax=[]  DivideOutMin=[]  DivideOutMax=[]  UdiffTsProdOutMin=[]  UdiffTsProdOutMax=[]  NTsProdOutMin=[]  NTsProdOutMax=[]  UintegralTsProdOutMin=[]  UintegralTsProdOutMax=[]  UngainTsProdOutMin=[]  UngainTsProdOutMax=[]  ClampingZeroOutDataTypeStr=Inherit: Inherit via back propagation  ClampingZeroOutMin=[]  ClampingZeroOutMax=[]  FilterDenConstantOutDataTypeStr=Inherit: Inherit via back propagation  FilterDenConstantOutMin=[]  FilterDenConstantOutMax=[]  PCopyOutDataTypeStr=Inherit: Inherit via back propagation  PCopyOutMin=[]  PCopyOutMax=[]  NCopyOutDataTypeStr=Inherit: Inherit via back propagation  NCopyOutMin=[]  NCopyOutMax=[]  IntegratorContinuousStateAttributes=''  IntegratorStateMustResolveToSignalObject=off  IntegratorRTWStateStorageClass=Auto  FilterContinuousStateAttributes=''  FilterStateMustResolveToSignalObject=off  FilterRTWStateStorageClass=Auto  ParallelPVariant=InternalParameters  IdealPVariant=Disabled  IVariant=InternalParameters  DVariant=Disabled  IntegratorVariant=Discrete  SatVariant=Enabled  AWVariant=DiscClampingParallel  PCopyVariant=Disabled  TRVariant=Disabled  FdbkBlocksVariant=Forward  IdealPFdbkVariant=Disabled  SatFdbkVariant=Disabled  DerivativeFilterVariant=Disabled  NVariant=Disabled  NCopyVariant=Disabled_SignalSpec  FilterICVariant=Disabled  IntegratorICVariant=InternalICs  ExternalResetVariant=Disabled  TRSumVariant=Passthrough  SumFdbkVariant=Disabled  SumVariant=Sum_PI  TsampFilterVariant=InternalTs  TsampNgainVariant=Passthrough  TsampIntegralVariant=Passthrough  ExternalSaturationOutDataTypeStr=Inherit: Same as second input
  Te_ref : Outport  SampleTime=5e-4
  wires:
  rpm_actual/1 -> Sum2/2
  Sum2/1 -> rpm_to_rad/s/1  "rpm_error"
  speed_controller/1 -> requested_torque_limited_to_0.1/1  "Te_req_for_speed_control"
  requested_torque_limited_to_0.1/1 -> Te_ref/1
  rpm_to_rad/s/1 -> speed_controller/1
  rpm_ref/1 -> Sum2/1
  Constant/1 -> ?

== system simulation_basic/Motor_Model/ADC Sampler ==
  In1 : Inport
  In2 : Inport  Port=2
  Trigger : TriggerPort  VariantControl=(inherit)  PortDimensions=1
  Unit Delay : UnitDelay  SampleTime=-1  HasFrameUpgradeWarning=on
  Unit Delay1 : UnitDelay  SampleTime=-1  HasFrameUpgradeWarning=on
  Out1 : Outport
  Out2 : Outport  Port=2
  wires:
  In2/1 -> Unit Delay1/1
  In1/1 -> Unit Delay/1
  Unit Delay/1 -> Out1/1
  Unit Delay1/1 -> Out2/1

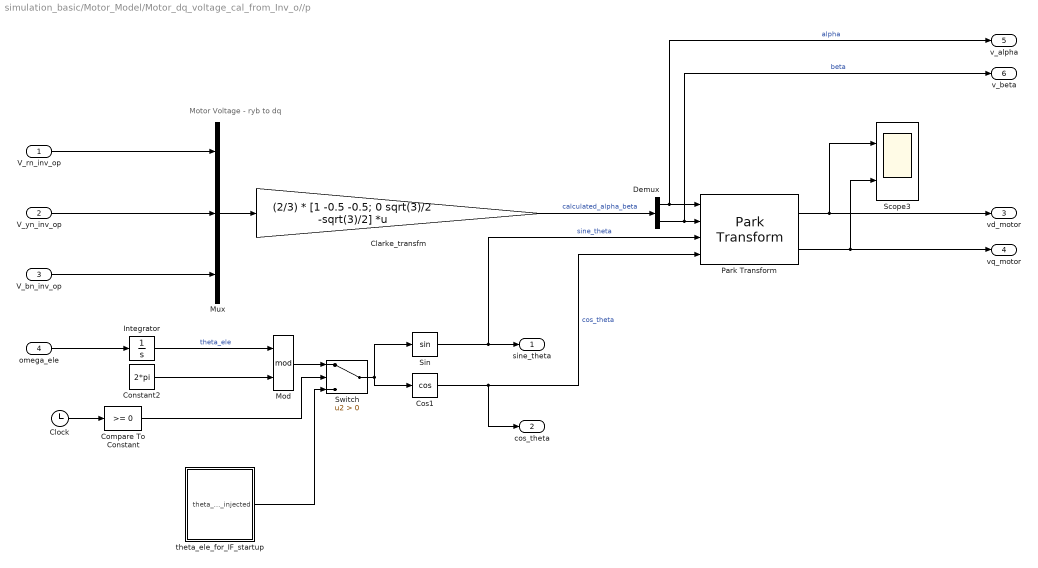
== system simulation_basic/Motor_Model/Motor_dq_voltage_cal_from_Inv_o//p ==
  note: Motor Voltage - ryb to dq
  V_rn_inv_op : Inport
  V_yn_inv_op : Inport  Port=2
  V_bn_inv_op : Inport  Port=3
  omega_ele : Inport  Port=4
  Clarke_transfm : Gain  Gain=(2/3) * [1 -0.5 -0.5; 0 sqrt(3)/2 -sqrt(3)/2]  Multiplication=Matrix(K*u)
  Clock : Clock
  Compare To Constant : simulink/Logic and Bit Operations/Compare To Constant  relop=>=  const=0  OutDataTypeStr=boolean
  Constant2 : Constant  Value=2*pi
  Cos1 : Trigonometry  Operator=cos
  Demux : Demux  Outputs=2
  Integrator : Integrator
  Mod : Math  Operator=mod
  Mux : Mux  Inputs=3
  Park Transform : mcbcontrolslib/Park Transform  AxisAlignment=D-axis
      settings: LibrarySourceBlock=mcbhdllib/Controls/Math Transforms/Park Transform
  Scope3 : Scope  NumInputPorts=2
  Sin : Trigonometry
  Switch : Switch  Criteria=u2 > Threshold  SaturateOnIntegerOverflow=off  InputSameDT=off
  theta_ele_for_IF_startup : Subsystem
  sine_theta : Outport
  cos_theta : Outport  Port=2
  vd_motor : Outport  Port=3
  vq_motor : Outport  Port=4
  v_alpha : Outport  Port=5
  v_beta : Outport  Port=6
  wires:
  Sin/1 -> sine_theta/1, Park Transform/3  "sine_theta"
  Constant2/1 -> Mod/2
  Cos1/1 -> cos_theta/1, Park Transform/4  "cos_theta"
  Demux/1 -> v_alpha/1, Park Transform/1  "alpha"
  Park Transform/2 -> Scope3/2, vq_motor/1
  Clarke_transfm/1 -> Demux/1  "calculated_alpha_beta"
  Integrator/1 -> Mod/1  "theta_ele"
  Demux/2 -> v_beta/1, Park Transform/2  "beta"
  Mux/1 -> Clarke_transfm/1
  Park Transform/1 -> vd_motor/1, Scope3/1
  V_bn_inv_op/1 -> Mux/3
  omega_ele/1 -> Integrator/1
  V_rn_inv_op/1 -> Mux/1
  V_yn_inv_op/1 -> Mux/2
  theta_ele_for_IF_startup/1(theta_ele_injected) -> Switch/3
  Mod/1 -> Switch/1
  Switch/1 -> Sin/1, Cos1/1
  Compare To Constant/1 -> Switch/2
  Clock/1 -> Compare To Constant/1

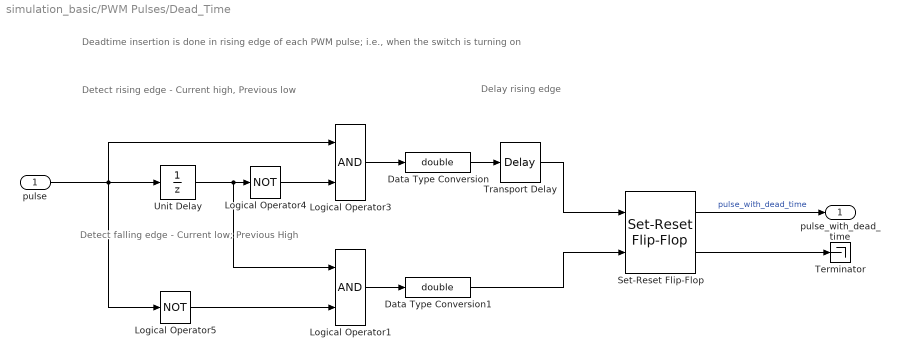
== system simulation_basic/PWM Pulses/Dead_Time ==
  note: Deadtime insertion is done in rising edge of each PWM pulse; i.e., when the switch is turning on
  note: Delay rising edge
  note: Detect falling edge - Current low; Previous High
  note: Detect rising edge - Current high, Previous low
  pulse : Inport
  Data Type Conversion : DataTypeConversion  OutDataTypeStr=double  SaturateOnIntegerOverflow=off  RndMeth=Floor
  Data Type Conversion1 : DataTypeConversion  OutDataTypeStr=double  SaturateOnIntegerOverflow=off  RndMeth=Floor
  Logical Operator1 : Logic  AllPortsSameDT=off  OutDataTypeStr=boolean
  Logical Operator3 : Logic  AllPortsSameDT=off  OutDataTypeStr=boolean
  Logical Operator4 : Logic  Operator=NOT  AllPortsSameDT=off  OutDataTypeStr=boolean
  Logical Operator5 : Logic  Operator=NOT  AllPortsSameDT=off  OutDataTypeStr=boolean
  Set-Reset Flip-Flop : eeGeneralControl/Set-Reset Flip-Flop  LabelModeActiveChoice=Discrete  UndefState=Set  Q0=0  Ts=-1
      settings: LibrarySourceBlock=ee_sl_lib/General Control/Set-Reset Flip-Flop
  Terminator : Terminator
  Transport Delay : TransportDelay  DelayTime=2e-6
  Unit Delay : UnitDelay  SampleTime=-1  HasFrameUpgradeWarning=on
  pulse_with_dead_time : Outport
  wires:
  Unit Delay/1 -> Logical Operator1/1, Logical Operator4/1
  pulse/1 -> Logical Operator5/1, Logical Operator3/1, Unit Delay/1
  Logical Operator5/1 -> Logical Operator1/2
  Logical Operator4/1 -> Logical Operator3/2
  Transport Delay/1 -> Set-Reset Flip-Flop/1
  Data Type Conversion/1 -> Transport Delay/1
  Logical Operator3/1 -> Data Type Conversion/1
  Data Type Conversion1/1 -> Set-Reset Flip-Flop/2
  Logical Operator1/1 -> Data Type Conversion1/1
  Set-Reset Flip-Flop/1 -> pulse_with_dead_time/1  "pulse_with_dead_time"
  Set-Reset Flip-Flop/2 -> Terminator/1

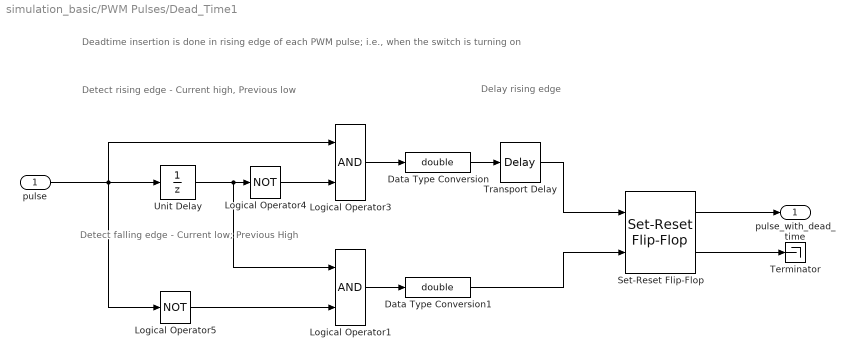
== system simulation_basic/PWM Pulses/Dead_Time1 ==
  note: Detect rising edge - Current high, Previous low
  note: Detect falling edge - Current low; Previous High
  note: Delay rising edge
  note: Deadtime insertion is done in rising edge of each PWM pulse; i.e., when the switch is turning on
  pulse : Inport
  Data Type Conversion : DataTypeConversion  OutDataTypeStr=double  SaturateOnIntegerOverflow=off  RndMeth=Floor
  Data Type Conversion1 : DataTypeConversion  OutDataTypeStr=double  SaturateOnIntegerOverflow=off  RndMeth=Floor
  Logical Operator1 : Logic  AllPortsSameDT=off  OutDataTypeStr=boolean
  Logical Operator3 : Logic  AllPortsSameDT=off  OutDataTypeStr=boolean
  Logical Operator4 : Logic  Operator=NOT  AllPortsSameDT=off  OutDataTypeStr=boolean
  Logical Operator5 : Logic  Operator=NOT  AllPortsSameDT=off  OutDataTypeStr=boolean
  Set-Reset Flip-Flop : eeGeneralControl/Set-Reset Flip-Flop  LabelModeActiveChoice=Discrete  UndefState=Set  Q0=0  Ts=-1
      settings: LibrarySourceBlock=ee_sl_lib/General Control/Set-Reset Flip-Flop
  Terminator : Terminator
  Transport Delay : TransportDelay  DelayTime=2e-6
  Unit Delay : UnitDelay  SampleTime=-1  HasFrameUpgradeWarning=on
  pulse_with_dead_time : Outport
  wires:
  Set-Reset Flip-Flop/2 -> Terminator/1
  Set-Reset Flip-Flop/1 -> pulse_with_dead_time/1
  Logical Operator1/1 -> Data Type Conversion1/1
  Data Type Conversion1/1 -> Set-Reset Flip-Flop/2
  Logical Operator3/1 -> Data Type Conversion/1
  Data Type Conversion/1 -> Transport Delay/1
  Transport Delay/1 -> Set-Reset Flip-Flop/1
  Logical Operator4/1 -> Logical Operator3/2
  Logical Operator5/1 -> Logical Operator1/2
  pulse/1 -> Unit Delay/1, Logical Operator3/1, Logical Operator5/1
  Unit Delay/1 -> Logical Operator4/1, Logical Operator1/1

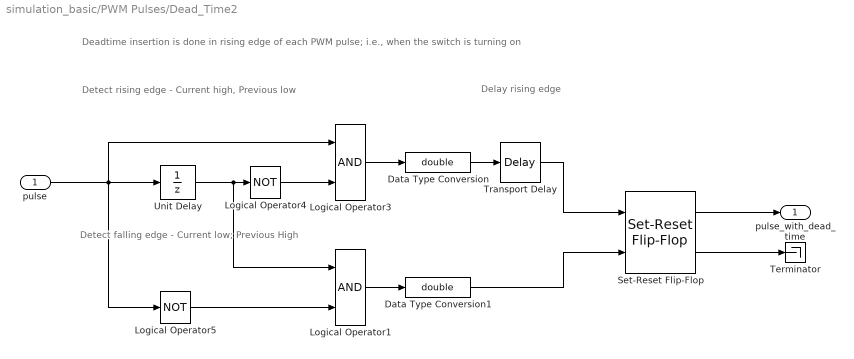
== system simulation_basic/PWM Pulses/Dead_Time2 ==
  note: Deadtime insertion is done in rising edge of each PWM pulse; i.e., when the switch is turning on
  note: Delay rising edge
  note: Detect falling edge - Current low; Previous High
  note: Detect rising edge - Current high, Previous low
  pulse : Inport
  Data Type Conversion : DataTypeConversion  OutDataTypeStr=double  SaturateOnIntegerOverflow=off  RndMeth=Floor
  Data Type Conversion1 : DataTypeConversion  OutDataTypeStr=double  SaturateOnIntegerOverflow=off  RndMeth=Floor
  Logical Operator1 : Logic  AllPortsSameDT=off  OutDataTypeStr=boolean
  Logical Operator3 : Logic  AllPortsSameDT=off  OutDataTypeStr=boolean
  Logical Operator4 : Logic  Operator=NOT  AllPortsSameDT=off  OutDataTypeStr=boolean
  Logical Operator5 : Logic  Operator=NOT  AllPortsSameDT=off  OutDataTypeStr=boolean
  Set-Reset Flip-Flop : eeGeneralControl/Set-Reset Flip-Flop  LabelModeActiveChoice=Discrete  UndefState=Set  Q0=0  Ts=-1
      settings: LibrarySourceBlock=ee_sl_lib/General Control/Set-Reset Flip-Flop
  Terminator : Terminator
  Transport Delay : TransportDelay  DelayTime=2e-6
  Unit Delay : UnitDelay  SampleTime=-1  HasFrameUpgradeWarning=on
  pulse_with_dead_time : Outport
  wires:
  Unit Delay/1 -> Logical Operator1/1, Logical Operator4/1
  pulse/1 -> Logical Operator5/1, Logical Operator3/1, Unit Delay/1
  Logical Operator5/1 -> Logical Operator1/2
  Logical Operator4/1 -> Logical Operator3/2
  Transport Delay/1 -> Set-Reset Flip-Flop/1
  Data Type Conversion/1 -> Transport Delay/1
  Logical Operator3/1 -> Data Type Conversion/1
  Data Type Conversion1/1 -> Set-Reset Flip-Flop/2
  Logical Operator1/1 -> Data Type Conversion1/1
  Set-Reset Flip-Flop/1 -> pulse_with_dead_time/1
  Set-Reset Flip-Flop/2 -> Terminator/1

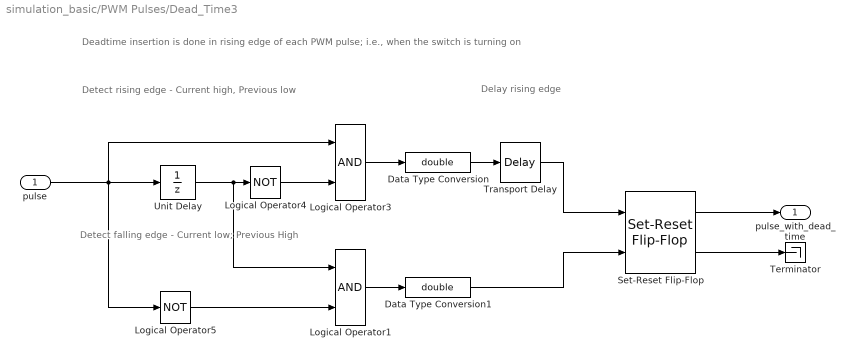
== system simulation_basic/PWM Pulses/Dead_Time3 ==
  note: Detect rising edge - Current high, Previous low
  note: Detect falling edge - Current low; Previous High
  note: Delay rising edge
  note: Deadtime insertion is done in rising edge of each PWM pulse; i.e., when the switch is turning on
  pulse : Inport
  Data Type Conversion : DataTypeConversion  OutDataTypeStr=double  SaturateOnIntegerOverflow=off  RndMeth=Floor
  Data Type Conversion1 : DataTypeConversion  OutDataTypeStr=double  SaturateOnIntegerOverflow=off  RndMeth=Floor
  Logical Operator1 : Logic  AllPortsSameDT=off  OutDataTypeStr=boolean
  Logical Operator3 : Logic  AllPortsSameDT=off  OutDataTypeStr=boolean
  Logical Operator4 : Logic  Operator=NOT  AllPortsSameDT=off  OutDataTypeStr=boolean
  Logical Operator5 : Logic  Operator=NOT  AllPortsSameDT=off  OutDataTypeStr=boolean
  Set-Reset Flip-Flop : eeGeneralControl/Set-Reset Flip-Flop  LabelModeActiveChoice=Discrete  UndefState=Set  Q0=0  Ts=-1
      settings: LibrarySourceBlock=ee_sl_lib/General Control/Set-Reset Flip-Flop
  Terminator : Terminator
  Transport Delay : TransportDelay  DelayTime=2e-6
  Unit Delay : UnitDelay  SampleTime=-1  HasFrameUpgradeWarning=on
  pulse_with_dead_time : Outport
  wires:
  Set-Reset Flip-Flop/2 -> Terminator/1
  Set-Reset Flip-Flop/1 -> pulse_with_dead_time/1
  Logical Operator1/1 -> Data Type Conversion1/1
  Data Type Conversion1/1 -> Set-Reset Flip-Flop/2
  Logical Operator3/1 -> Data Type Conversion/1
  Data Type Conversion/1 -> Transport Delay/1
  Transport Delay/1 -> Set-Reset Flip-Flop/1
  Logical Operator4/1 -> Logical Operator3/2
  Logical Operator5/1 -> Logical Operator1/2
  pulse/1 -> Unit Delay/1, Logical Operator3/1, Logical Operator5/1
  Unit Delay/1 -> Logical Operator4/1, Logical Operator1/1

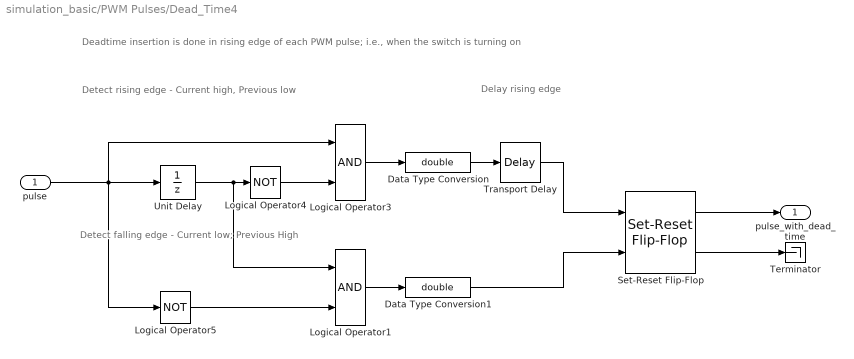
== system simulation_basic/PWM Pulses/Dead_Time4 ==
  note: Deadtime insertion is done in rising edge of each PWM pulse; i.e., when the switch is turning on
  note: Delay rising edge
  note: Detect falling edge - Current low; Previous High
  note: Detect rising edge - Current high, Previous low
  pulse : Inport
  Data Type Conversion : DataTypeConversion  OutDataTypeStr=double  SaturateOnIntegerOverflow=off  RndMeth=Floor
  Data Type Conversion1 : DataTypeConversion  OutDataTypeStr=double  SaturateOnIntegerOverflow=off  RndMeth=Floor
  Logical Operator1 : Logic  AllPortsSameDT=off  OutDataTypeStr=boolean
  Logical Operator3 : Logic  AllPortsSameDT=off  OutDataTypeStr=boolean
  Logical Operator4 : Logic  Operator=NOT  AllPortsSameDT=off  OutDataTypeStr=boolean
  Logical Operator5 : Logic  Operator=NOT  AllPortsSameDT=off  OutDataTypeStr=boolean
  Set-Reset Flip-Flop : eeGeneralControl/Set-Reset Flip-Flop  LabelModeActiveChoice=Discrete  UndefState=Set  Q0=0  Ts=-1
      settings: LibrarySourceBlock=ee_sl_lib/General Control/Set-Reset Flip-Flop
  Terminator : Terminator
  Transport Delay : TransportDelay  DelayTime=2e-6
  Unit Delay : UnitDelay  SampleTime=-1  HasFrameUpgradeWarning=on
  pulse_with_dead_time : Outport
  wires:
  Unit Delay/1 -> Logical Operator1/1, Logical Operator4/1
  pulse/1 -> Logical Operator5/1, Logical Operator3/1, Unit Delay/1
  Logical Operator5/1 -> Logical Operator1/2
  Logical Operator4/1 -> Logical Operator3/2
  Transport Delay/1 -> Set-Reset Flip-Flop/1
  Data Type Conversion/1 -> Transport Delay/1
  Logical Operator3/1 -> Data Type Conversion/1
  Data Type Conversion1/1 -> Set-Reset Flip-Flop/2
  Logical Operator1/1 -> Data Type Conversion1/1
  Set-Reset Flip-Flop/1 -> pulse_with_dead_time/1
  Set-Reset Flip-Flop/2 -> Terminator/1

== system simulation_basic/PWM Pulses/Dead_Time5 ==
  note: Detect rising edge - Current high, Previous low
  note: Detect falling edge - Current low; Previous High
  note: Delay rising edge
  note: Deadtime insertion is done in rising edge of each PWM pulse; i.e., when the switch is turning on
  pulse : Inport
  Data Type Conversion : DataTypeConversion  OutDataTypeStr=double  SaturateOnIntegerOverflow=off  RndMeth=Floor
  Data Type Conversion1 : DataTypeConversion  OutDataTypeStr=double  SaturateOnIntegerOverflow=off  RndMeth=Floor
  Logical Operator1 : Logic  AllPortsSameDT=off  OutDataTypeStr=boolean
  Logical Operator3 : Logic  AllPortsSameDT=off  OutDataTypeStr=boolean
  Logical Operator4 : Logic  Operator=NOT  AllPortsSameDT=off  OutDataTypeStr=boolean
  Logical Operator5 : Logic  Operator=NOT  AllPortsSameDT=off  OutDataTypeStr=boolean
  Set-Reset Flip-Flop : eeGeneralControl/Set-Reset Flip-Flop  LabelModeActiveChoice=Discrete  UndefState=Set  Q0=0  Ts=-1
      settings: LibrarySourceBlock=ee_sl_lib/General Control/Set-Reset Flip-Flop
  Terminator : Terminator
  Transport Delay : TransportDelay  DelayTime=2e-6
  Unit Delay : UnitDelay  SampleTime=-1  HasFrameUpgradeWarning=on
  pulse_with_dead_time : Outport
  wires:
  Set-Reset Flip-Flop/2 -> Terminator/1
  Set-Reset Flip-Flop/1 -> pulse_with_dead_time/1
  Logical Operator1/1 -> Data Type Conversion1/1
  Data Type Conversion1/1 -> Set-Reset Flip-Flop/2
  Logical Operator3/1 -> Data Type Conversion/1
  Data Type Conversion/1 -> Transport Delay/1
  Transport Delay/1 -> Set-Reset Flip-Flop/1
  Logical Operator4/1 -> Logical Operator3/2
  Logical Operator5/1 -> Logical Operator1/2
  pulse/1 -> Unit Delay/1, Logical Operator3/1, Logical Operator5/1
  Unit Delay/1 -> Logical Operator4/1, Logical Operator1/1

== system simulation_basic/current_controller/omega_ele_injected_IF_startup ==
  Constant : Constant  Value=motor.pp
  Product : Product
  Ramp : simulink/Sources/Ramp  slope=50  start=0.2  InitialOutput=0
  rpm_to_rad/s_mech : Gain  Gain=2*pi/60
  omega_ele_injected : Outport
  wires:
  Product/1 -> omega_ele_injected/1  "omega_ele_injected"
  rpm_to_rad/s_mech/1 -> Product/1
  Constant/1 -> Product/2
  Ramp/1 -> rpm_to_rad/s_mech/1  "rpm_for_IF"

== system simulation_basic/Motor_Model/Motor_dq_voltage_cal_from_Inv_o//p/theta_ele_for_IF_startup ==
  Constant : Constant  Value=motor.pp
  Integrator : Integrator  WrapState=on  WrappedStateUpperValue=2*pi  WrappedStateLowerValue=0
  Product : Product
  Ramp : simulink/Sources/Ramp  slope=50  start=0.2  InitialOutput=0
  rpm_to_rad/s_mech : Gain  Gain=2*pi/60
  theta_ele_injected : Outport
  wires:
  Product/1 -> Integrator/1  "omega_ele"
  Integrator/1 -> theta_ele_injected/1  "theta_ele_injected"
  rpm_to_rad/s_mech/1 -> Product/1
  Constant/1 -> Product/2
  Ramp/1 -> rpm_to_rad/s_mech/1  "rpm_for_IF"

== matlab function simulation_basic/MATLAB Function1 ==
  data: u input; y output
function y = fcn(u)
% Assuming 'signal' is your input vector or value
noise_percentage = 0.10; % 10%
%rand(noise_percentage);
y = u + (u .* randn(size(u)) * noise_percentage);
%y = u + (u * noise_percentage);
